simulink model "test_L_detector"  (Simulink 7.6)
settings: Solver=FixedStepDiscrete  StartTime=0.0  StopTime=0  RelTol=1e-3
values from neighbouring files (symbols this model uses):
  Forward_Camera_Dimensions = [640 480]    [VisionConstants.m]
  Iter_Segment_Thresh = 60    [VisionConstants.m]
  Scale_Forward_B = 1    [VisionConstants.m]
  Scale_Forward_G = 1    [VisionConstants.m]
  Scale_Forward_H = .8    (= 0.8)    [VisionConstants.m]
  Scale_Forward_R = 1    [VisionConstants.m]
  Scale_Forward_S = 1    [VisionConstants.m]
  Scale_Forward_V = 2    [VisionConstants.m]
undefined symbols (not defined in the file or in its folder): black_al, black_au, black_bl, black_bu, blue_al, blue_au, blue_bl, blue_bu, Forward_Fov, gray, green_al, green_au, green_bl, green_bu, orange_al, orange_au, orange_bl, orange_bu, Rec, red_al, red_au, red_bl, red_bu, SDTV, white_al, white_au, white_bl, white_bu, yellow_al, yellow_au, yellow_bl, yellow_bu
libraries: vipconversions x4, vipgeotforms x3, viptextngfix x2, vipsnks x2, viptransforms x2, vipanalysis x1, vipsrcs x1
(part 1 of 2)
settings Model: Creator=Thing 1  LastModifiedBy=auvt
settings RTWCC: TargetLang=C++

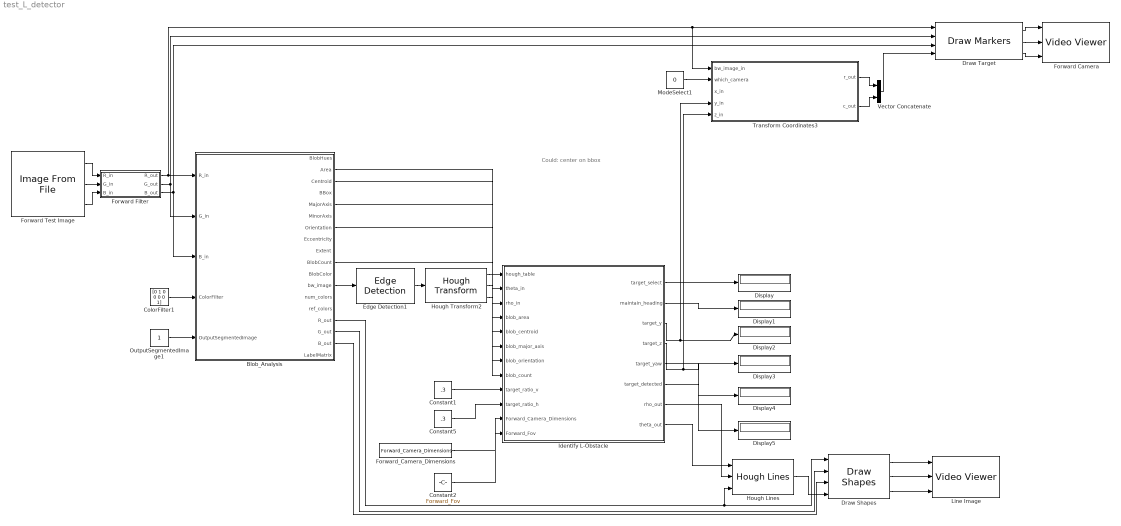
== system test_L_detector ==
  note: Could: center on bbox
  Blob_Analysis : Subsystem
  ColorFilter1 : Constant  Value=[0 1 0 0 0 0 1]  SampleTime=-1
  Constant1 : Constant  Value=.3  SampleTime=-1
  Constant2 : Constant  Value=Forward_Fov  SampleTime=-1
  Constant5 : Constant  Value=.3  SampleTime=-1
  Display{,1..5} (6 alike) : Display
  Draw Shapes : viptextngfix/Draw Shapes  DialogController=vipDDGCreate  DialogControllerArgs=DataTag3  shape=Lines  fill=off  fillClrSource=Specify via dialog  display=Black  intensity=200  color=[200 255 100]  opacity=0.6  viewport=Entire image  antialiasing=off  inType=Obsolete  imagePorts=Separate color signals  prodOutputMode=Binary point scaling  prodOutputWordLength=32  prodOutputFracLength=14  memoryMode=Specify word length  memoryWordLength=16  memoryFracLength=15  roundingMode=Floor  overflowMode=off
  Draw Target : viptextngfix/Draw Markers  DialogController=vipDDGCreate  DialogControllerArgs=DataTag4  shape=X-mark  size=7  fill=off  fillClrSource=Specify via dialog  display=User-specified value  intensity=200  color=[1 0 0]  opacity=0.6  viewport=Entire image  antialiasing=off  inType=Obsolete  imagePorts=Separate color signals  prodOutputMode=Binary point scaling  prodOutputWordLength=32  prodOutputFracLength=14  memoryMode=Specify word length  memoryWordLength=16  memoryFracLength=15  roundingMode=Floor  overflowMode=off
  Edge Detection1 : vipanalysis/Edge Detection  DialogController=vipDDGCreate  DialogControllerArgs=DataTag5  method=Sobel  outputType=Binary image  userDefinedThreshold=off  thresholdSource=Specify via dialog  threshold=20  thresholdTuning=3  edgeThinning=on  threshold_canny=[0.25 0.60]  autoPercent=70  sigma=1  roundingMode=Floor  overflowMode=off
  Forward Camera : vipsnks/Video Viewer  DialogControllerArgs=DataTag7  inputType=Obsolete7b  imagePorts=Separate color signals  useColorMap=off  colormapValue=gray(256)  specRange=off  minInputVal=0  maxInputVal=255  FigPos=[1161 458 276 283]  AxisZoom=on  trueSizedOnce=off  OpenAtMdlStart=on
  Forward Filter : Subsystem
  Forward Test Image : vipsrcs/Image From File  Tag=vipblks_nd  DialogController=vipDDGCreate  DialogControllerArgs=DataTag8  SystemSampleTime=-1  FileName=/home/auvt/auvc/src/vision/Test_Images/L1.PNG  imagePorts=Separate color signals  Ts=-1  ImageDataType=double  Signed=on  WordLength=16  sdImageDataType=uint(8)  FractionLengthMode=User-defined  FractionLength=15  OutPortLabels=R|G|B
  Forward_Camera_Dimensions : Constant  Value=Forward_Camera_Dimensions  SampleTime=-1
  Hough Lines : viptransforms/Hough Lines  DialogController=vipDDGCreate  DialogControllerArgs=DataTag9  sineCompMethod=Trigonometric function  thetaRes=pi/180  firstCoeffMode=Specify word length  firstCoeffWordLength=16  firstCoeffFracLength=15  prodOutputMode=Binary point scaling  prodOutputWordLength=32  prodOutputFracLength=16  roundingMode=Nearest  overflowMode=on
  Hough Transform2 : viptransforms/Hough Transform  DialogController=vipDDGCreate  DialogControllerArgs=DataTag10  theta_res=pi/180  rho_res=1  out_theta_rho=on  outdtmode=double  firstCoeffMode=Binary point scaling  firstCoeffWordLength=16  firstCoeffFracLength=14  secondCoeffMode=Binary point scaling  secondCoeffWordLength=32  secondCoeffFracLength=16  outputMode=Binary point scaling  outputWordLength=16  outputFracLength=0  accumMode=Binary point scaling  accumWordLength=32  accumFracLength=20  prodOutputMode=Binary point scaling  prodOutputWordLength=32  prodOutputFracLength=20  memoryMode=Binary point scaling  memoryWordLength=32  memoryFracLength=16  roundingMode=Nearest  overflowMode=on
  Identify L-Obstacle : Stateflow chart  TreatAsAtomicUnit=on  SystemSampleTime=[1/30 0]
  Line Image : vipsnks/Video Viewer  DialogControllerArgs=DataTag12  inputType=Obsolete7b  imagePorts=Separate color signals  useColorMap=off  colormapValue=gray(256)  specRange=off  minInputVal=0  maxInputVal=255  FigPos=[1163 861 274 294]  AxisZoom=on  trueSizedOnce=off  OpenAtMdlStart=on
  ModeSelect1 : Constant  Value=0  SampleTime=-1
  OutputSegmentedImage1 : Constant  SampleTime=-1
  Transform Coordinates3 : Stateflow chart  TreatAsAtomicUnit=on  SystemSampleTime=[1/30 0]
  Vector Concatenate : Concatenate  Mode=Multidimensional array
  wires:
  Forward Test Image/1 -> Forward Filter/1(R_in)
  Forward Test Image/3 -> Forward Filter/3(B_in)
  Vector Concatenate/1 -> Draw Target/4
  Draw Target/2 -> Forward Camera/2
  Draw Target/1 -> Forward Camera/1
  Draw Target/3 -> Forward Camera/3
  Forward Filter/1(R_out) -> Draw Target/1, Transform Coordinates3/1(bw_image_in), Blob_Analysis/1(R_in)
  Forward Filter/2(G_out) -> Draw Target/2, Blob_Analysis/2(G_in)
  Forward Filter/3(B_out) -> Draw Target/3, Blob_Analysis/3(B_in)
  Forward Test Image/2 -> Forward Filter/2(G_in)
  ModeSelect1/1 -> Transform Coordinates3/2(which_camera)
  Transform Coordinates3/1(r_out) -> Vector Concatenate/1
  Transform Coordinates3/2(c_out) -> Vector Concatenate/2
  OutputSegmentedImage1/1 -> Blob_Analysis/5(OutputSegmentedImage)
  ColorFilter1/1 -> Blob_Analysis/4(ColorFilter)
  Edge Detection1/1 -> Hough Transform2/1
  Blob_Analysis/12(bw_image) -> Edge Detection1/1
  Hough Transform2/1 -> Identify L-Obstacle/1(hough_table)
  Hough Transform2/2 -> Identify L-Obstacle/2(theta_in)
  Hough Transform2/3 -> Identify L-Obstacle/3(rho_in)
  Blob_Analysis/2(Area) -> Identify L-Obstacle/4(blob_area)
  Blob_Analysis/3(Centroid) -> Identify L-Obstacle/5(blob_centroid)
  Blob_Analysis/5(MajorAxis) -> Identify L-Obstacle/6(blob_major_axis)
  Blob_Analysis/7(Orientation) -> Identify L-Obstacle/7(blob_orientation)
  Blob_Analysis/10(BlobCount) -> Identify L-Obstacle/8(blob_count)
  Constant1/1 -> Identify L-Obstacle/9(target_ratio_v)
  Constant5/1 -> Identify L-Obstacle/10(target_ratio_h)
  Forward_Camera_Dimensions/1 -> Identify L-Obstacle/11(Forward_Camera_Dimensions)
  Constant2/1 -> Identify L-Obstacle/12(Forward_Fov)
  Identify L-Obstacle/3(target_y) -> Display2/1, Transform Coordinates3/4(y_in)
  Identify L-Obstacle/1(target_select) -> Display/1
  Identify L-Obstacle/2(maintain_heading) -> Display1/1
  Identify L-Obstacle/4(target_z) -> Display3/1, Transform Coordinates3/5(z_in)
  Identify L-Obstacle/5(target_yaw) -> Display4/1
  Identify L-Obstacle/6(target_detected) -> Display5/1
  Draw Shapes/1 -> Line Image/1
  Draw Shapes/2 -> Line Image/2
  Draw Shapes/3 -> Line Image/3
  Hough Lines/1 -> Draw Shapes/4
  Blob_Analysis/15(R_out) -> Draw Shapes/1, Hough Lines/3
  Blob_Analysis/16(G_out) -> Draw Shapes/2
  Blob_Analysis/17(B_out) -> Draw Shapes/3
  Identify L-Obstacle/8(theta_out) -> Hough Lines/1
  Identify L-Obstacle/7(rho_out) -> Hough Lines/2

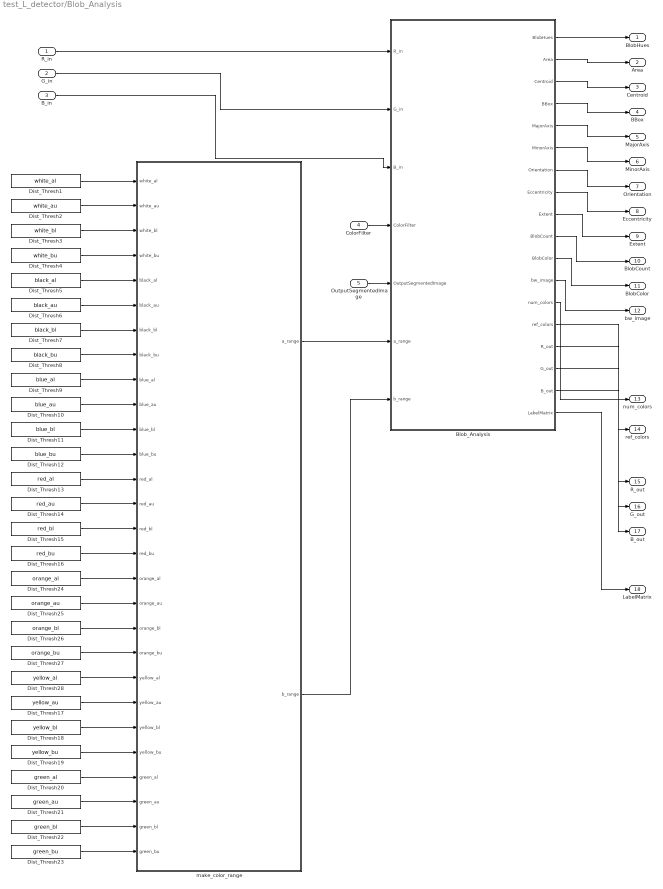
== system test_L_detector/Blob_Analysis ==
  R_in : Inport
  G_in : Inport  Port=2
  B_in : Inport  Port=3
  ColorFilter : Inport  Port=4
  OutputSegmentedImage : Inport  Port=5
  Blob_Analysis : Subsystem  TreatAsAtomicUnit=on
  Dist_Thresh1 : Constant  Value=white_al  SampleTime=-1
  Dist_Thresh10 : Constant  Value=blue_au  SampleTime=-1
  Dist_Thresh11 : Constant  Value=blue_bl  SampleTime=-1
  Dist_Thresh12 : Constant  Value=blue_bu  SampleTime=-1
  Dist_Thresh13 : Constant  Value=red_al  SampleTime=-1
  Dist_Thresh14 : Constant  Value=red_au  SampleTime=-1
  Dist_Thresh15 : Constant  Value=red_bl  SampleTime=-1
  Dist_Thresh16 : Constant  Value=red_bu  SampleTime=-1
  Dist_Thresh17 : Constant  Value=yellow_au  SampleTime=-1
  Dist_Thresh18 : Constant  Value=yellow_bl  SampleTime=-1
  Dist_Thresh19 : Constant  Value=yellow_bu  SampleTime=-1
  Dist_Thresh2 : Constant  Value=white_au  SampleTime=-1
  Dist_Thresh20 : Constant  Value=green_al  SampleTime=-1
  Dist_Thresh21 : Constant  Value=green_au  SampleTime=-1
  Dist_Thresh22 : Constant  Value=green_bl  SampleTime=-1
  Dist_Thresh23 : Constant  Value=green_bu  SampleTime=-1
  Dist_Thresh24 : Constant  Value=orange_al  SampleTime=-1
  Dist_Thresh25 : Constant  Value=orange_au  SampleTime=-1
  Dist_Thresh26 : Constant  Value=orange_bl  SampleTime=-1
  Dist_Thresh27 : Constant  Value=orange_bu  SampleTime=-1
  Dist_Thresh28 : Constant  Value=yellow_al  SampleTime=-1
  Dist_Thresh3 : Constant  Value=white_bl  SampleTime=-1
  Dist_Thresh4 : Constant  Value=white_bu  SampleTime=-1
  Dist_Thresh5 : Constant  Value=black_al  SampleTime=-1
  Dist_Thresh6 : Constant  Value=black_au  SampleTime=-1
  Dist_Thresh7 : Constant  Value=black_bl  SampleTime=-1
  Dist_Thresh8 : Constant  Value=black_bu  SampleTime=-1
  Dist_Thresh9 : Constant  Value=blue_al  SampleTime=-1
  make_color_range : Stateflow chart  TreatAsAtomicUnit=on
  BlobHues : Outport
  Area : Outport  Port=2
  Centroid : Outport  Port=3
  BBox : Outport  Port=4
  MajorAxis : Outport  Port=5
  MinorAxis : Outport  Port=6
  Orientation : Outport  Port=7
  Eccentricity : Outport  Port=8
  Extent : Outport  Port=9
  BlobCount : Outport  Port=10
  BlobColor : Outport  Port=11
  bw_image : Outport  Port=12
  num_colors : Outport  Port=13
  ref_colors : Outport  Port=14
  R_out : Outport  Port=15
  G_out : Outport  Port=16
  B_out : Outport  Port=17
  LabelMatrix : Outport  Port=18
  wires:
  Dist_Thresh23/1 -> make_color_range/28(green_bu)
  Dist_Thresh22/1 -> make_color_range/27(green_bl)
  Dist_Thresh1/1 -> make_color_range/1(white_al)
  Dist_Thresh18/1 -> make_color_range/23(yellow_bl)
  Dist_Thresh19/1 -> make_color_range/24(yellow_bu)
  Dist_Thresh20/1 -> make_color_range/25(green_al)
  Dist_Thresh17/1 -> make_color_range/22(yellow_au)
  Dist_Thresh28/1 -> make_color_range/21(yellow_al)
  Dist_Thresh21/1 -> make_color_range/26(green_au)
  Dist_Thresh27/1 -> make_color_range/20(orange_bu)
  Dist_Thresh26/1 -> make_color_range/19(orange_bl)
  Dist_Thresh25/1 -> make_color_range/18(orange_au)
  Dist_Thresh24/1 -> make_color_range/17(orange_al)
  Dist_Thresh16/1 -> make_color_range/16(red_bu)
  Dist_Thresh15/1 -> make_color_range/15(red_bl)
  Dist_Thresh14/1 -> make_color_range/14(red_au)
  Dist_Thresh13/1 -> make_color_range/13(red_al)
  Dist_Thresh12/1 -> make_color_range/12(blue_bu)
  Dist_Thresh11/1 -> make_color_range/11(blue_bl)
  Dist_Thresh10/1 -> make_color_range/10(blue_au)
  Dist_Thresh9/1 -> make_color_range/9(blue_al)
  Dist_Thresh8/1 -> make_color_range/8(black_bu)
  Dist_Thresh2/1 -> make_color_range/2(white_au)
  Dist_Thresh3/1 -> make_color_range/3(white_bl)
  Dist_Thresh4/1 -> make_color_range/4(white_bu)
  Dist_Thresh5/1 -> make_color_range/5(black_al)
  Dist_Thresh6/1 -> make_color_range/6(black_au)
  Dist_Thresh7/1 -> make_color_range/7(black_bl)
  R_in/1 -> Blob_Analysis/1(R_in)
  G_in/1 -> Blob_Analysis/2(G_in)
  B_in/1 -> Blob_Analysis/3(B_in)
  make_color_range/1(a_range) -> Blob_Analysis/6(a_range)
  make_color_range/2(b_range) -> Blob_Analysis/7(b_range)
  OutputSegmentedImage/1 -> Blob_Analysis/5(OutputSegmentedImage)
  ColorFilter/1 -> Blob_Analysis/4(ColorFilter)
  Blob_Analysis/1(BlobHues) -> BlobHues/1
  Blob_Analysis/2(Area) -> Area/1
  Blob_Analysis/3(Centroid) -> Centroid/1
  Blob_Analysis/4(BBox) -> BBox/1
  Blob_Analysis/5(MajorAxis) -> MajorAxis/1
  Blob_Analysis/6(MinorAxis) -> MinorAxis/1
  Blob_Analysis/7(Orientation) -> Orientation/1
  Blob_Analysis/8(Eccentricity) -> Eccentricity/1
  Blob_Analysis/9(Extent) -> Extent/1
  Blob_Analysis/10(BlobCount) -> BlobCount/1
  Blob_Analysis/11(BlobColor) -> BlobColor/1
  Blob_Analysis/12(bw_image) -> bw_image/1
  Blob_Analysis/13(num_colors) -> num_colors/1
  Blob_Analysis/14(ref_colors) -> ref_colors/1
  Blob_Analysis/15(R_out) -> R_out/1
  Blob_Analysis/16(G_out) -> G_out/1
  Blob_Analysis/17(B_out) -> B_out/1
  Blob_Analysis/18(LabelMatrix) -> LabelMatrix/1

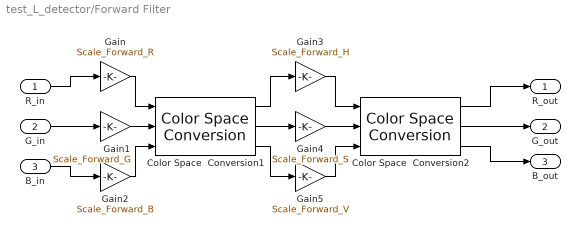
== system test_L_detector/Forward Filter ==
  R_in : Inport  PortDimensions=Forward_Camera_Dimensions
  G_in : Inport  Port=2  PortDimensions=Forward_Camera_Dimensions
  B_in : Inport  Port=3  PortDimensions=Forward_Camera_Dimensions
  Color Space  Conversion1 : vipconversions/Color Space  Conversion  conversion=Obsolete  conversionActive=R'G'B' to HSV  wp_str=D50  rec=Rec. 601 (SDTV)  sys=1125/60/2:1  imagePorts=Separate color signals
  Color Space  Conversion2 : vipconversions/Color Space  Conversion  conversion=Obsolete  conversionActive=HSV to R'G'B'  wp_str=D50  rec=Rec. 601 (SDTV)  sys=1125/60/2:1  imagePorts=Separate color signals
  Gain : Gain  Gain=Scale_Forward_R
  Gain1 : Gain  Gain=Scale_Forward_G
  Gain2 : Gain  Gain=Scale_Forward_B
  Gain3 : Gain  Gain=Scale_Forward_H
  Gain4 : Gain  Gain=Scale_Forward_S
  Gain5 : Gain  Gain=Scale_Forward_V
  R_out : Outport  OutDataTypeStr=double
  G_out : Outport  Port=2  OutDataTypeStr=double
  B_out : Outport  Port=3  OutDataTypeStr=double
  wires:
  R_in/1 -> Gain/1
  G_in/1 -> Gain1/1
  B_in/1 -> Gain2/1
  Gain/1 -> Color Space  Conversion1/1
  Gain1/1 -> Color Space  Conversion1/2
  Gain2/1 -> Color Space  Conversion1/3
  Color Space  Conversion1/1 -> Gain3/1
  Color Space  Conversion1/2 -> Gain4/1
  Color Space  Conversion1/3 -> Gain5/1
  Gain3/1 -> Color Space  Conversion2/1
  Gain4/1 -> Color Space  Conversion2/2
  Gain5/1 -> Color Space  Conversion2/3
  Color Space  Conversion2/1 -> R_out/1
  Color Space  Conversion2/2 -> G_out/1
  Color Space  Conversion2/3 -> B_out/1

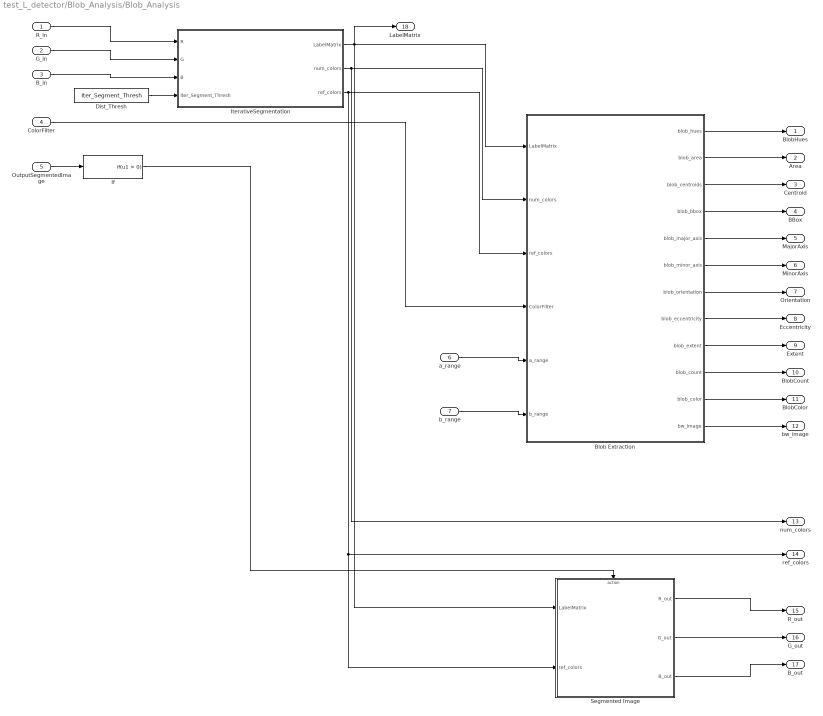
== system test_L_detector/Blob_Analysis/Blob_Analysis ==
  R_in : Inport
  G_in : Inport  Port=2
  B_in : Inport  Port=3
  ColorFilter : Inport  Port=4
  OutputSegmentedImage : Inport  Port=5
  a_range : Inport  Port=6
  b_range : Inport  Port=7
  Blob Extraction : Stateflow chart  TreatAsAtomicUnit=on
  Dist_Thresh : Constant  Value=Iter_Segment_Thresh  SampleTime=-1
  If : If  ShowElse=off
  IterativeSegmentation : Subsystem
      settings: UndoDeleteFcn=Stateflow.SLINSF.SimulinkMan.restorePreDeleteFcn  PreDeleteFcn=Stateflow.SLINSF.SimulinkMan.removePreDeleteFcn
  Segmented Image : Subsystem  TreatAsAtomicUnit=on
  BlobHues : Outport
  Area : Outport  Port=2
  Centroid : Outport  Port=3
  BBox : Outport  Port=4
  MajorAxis : Outport  Port=5
  MinorAxis : Outport  Port=6
  Orientation : Outport  Port=7
  Eccentricity : Outport  Port=8
  Extent : Outport  Port=9
  BlobCount : Outport  Port=10
  BlobColor : Outport  Port=11
  bw_image : Outport  Port=12
  num_colors : Outport  Port=13
  ref_colors : Outport  Port=14
  R_out : Outport  Port=15
  G_out : Outport  Port=16
  B_out : Outport  Port=17
  LabelMatrix : Outport  Port=18
  wires:
  Blob Extraction/12(bw_image) -> bw_image/1
  Blob Extraction/10(blob_count) -> BlobCount/1
  Blob Extraction/9(blob_extent) -> Extent/1
  Blob Extraction/8(blob_eccentricity) -> Eccentricity/1
  Blob Extraction/7(blob_orientation) -> Orientation/1
  Blob Extraction/6(blob_minor_axis) -> MinorAxis/1
  Blob Extraction/5(blob_major_axis) -> MajorAxis/1
  Blob Extraction/4(blob_bbox) -> BBox/1
  Blob Extraction/3(blob_centroids) -> Centroid/1
  Blob Extraction/2(blob_area) -> Area/1
  Blob Extraction/1(blob_hues) -> BlobHues/1
  ColorFilter/1 -> Blob Extraction/4(ColorFilter)
  a_range/1 -> Blob Extraction/5(a_range)
  b_range/1 -> Blob Extraction/6(b_range)
  IterativeSegmentation/1(LabelMatrix) -> Blob Extraction/1(LabelMatrix), Segmented Image/1(LabelMatrix), LabelMatrix/1
  IterativeSegmentation/2(num_colors) -> Blob Extraction/2(num_colors), num_colors/1
  IterativeSegmentation/3(ref_colors) -> Blob Extraction/3(ref_colors), Segmented Image/2(ref_colors), ref_colors/1
  Dist_Thresh/1 -> IterativeSegmentation/4(Iter_Segment_Thresh)
  R_in/1 -> IterativeSegmentation/1(R)
  G_in/1 -> IterativeSegmentation/2(G)
  B_in/1 -> IterativeSegmentation/3(B)
  If/1 -> Segmented Image/Action
  OutputSegmentedImage/1 -> If/1
  Segmented Image/1(R_out) -> R_out/1
  Segmented Image/2(G_out) -> G_out/1
  Segmented Image/3(B_out) -> B_out/1
  Blob Extraction/11(blob_color) -> BlobColor/1

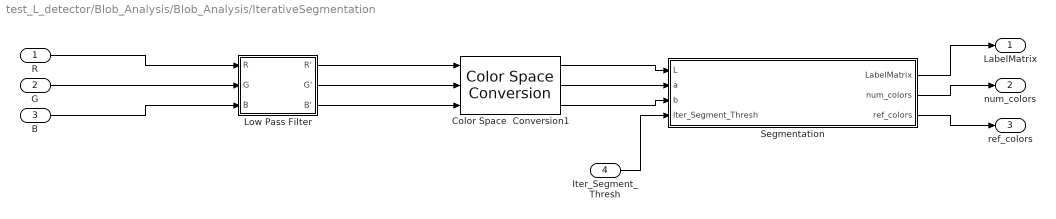
== system test_L_detector/Blob_Analysis/Blob_Analysis/IterativeSegmentation ==
  R : Inport
  G : Inport  Port=2
  B : Inport  Port=3
  Iter_Segment_Thresh : Inport  Port=4
  Color Space  Conversion1 : vipconversions/Color Space  Conversion  conversion=Obsolete  conversionActive=sR'G'B' to L*a*b*  wp_str=D50  rec=Rec. 601 (SDTV)  sys=1125/60/2:1  imagePorts=Separate color signals
  Low Pass Filter : Subsystem
  Segmentation : Subsystem
  LabelMatrix : Outport
  num_colors : Outport  Port=2
  ref_colors : Outport  Port=3
  wires:
  Low Pass Filter/3(B') -> Color Space  Conversion1/3
  Low Pass Filter/2(G') -> Color Space  Conversion1/2
  Low Pass Filter/1(R') -> Color Space  Conversion1/1
  Color Space  Conversion1/3 -> Segmentation/3(b)
  Color Space  Conversion1/2 -> Segmentation/2(a)
  Color Space  Conversion1/1 -> Segmentation/1(L)
  R/1 -> Low Pass Filter/1(R)
  G/1 -> Low Pass Filter/2(G)
  B/1 -> Low Pass Filter/3(B)
  Segmentation/1(LabelMatrix) -> LabelMatrix/1
  Segmentation/2(num_colors) -> num_colors/1
  Segmentation/3(ref_colors) -> ref_colors/1
  Iter_Segment_Thresh/1 -> Segmentation/4(Iter_Segment_Thresh)

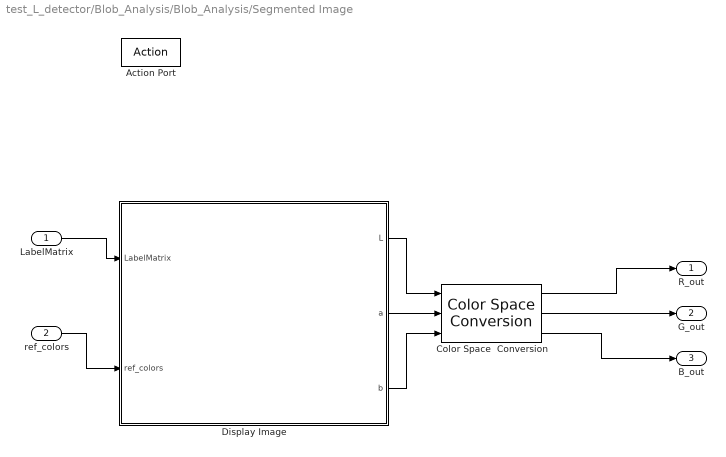
== system test_L_detector/Blob_Analysis/Blob_Analysis/Segmented Image ==
  LabelMatrix : Inport
  ref_colors : Inport  Port=2
  Action Port : ActionPort  ActionType=then
  Color Space  Conversion : vipconversions/Color Space  Conversion  conversion=Obsolete  conversionActive=L*a*b* to sR'G'B'  wp_str=D65  rec=Rec. 601 (SDTV)  sys=1125/60/2:1  imagePorts=Separate color signals
  Display Image : Stateflow chart  TreatAsAtomicUnit=on
  R_out : Outport
  G_out : Outport  Port=2
  B_out : Outport  Port=3
  wires:
  LabelMatrix/1 -> Display Image/1(LabelMatrix)
  ref_colors/1 -> Display Image/2(ref_colors)
  Display Image/1(L) -> Color Space  Conversion/1
  Display Image/2(a) -> Color Space  Conversion/2
  Display Image/3(b) -> Color Space  Conversion/3
  Color Space  Conversion/1 -> R_out/1
  Color Space  Conversion/2 -> G_out/1
  Color Space  Conversion/3 -> B_out/1

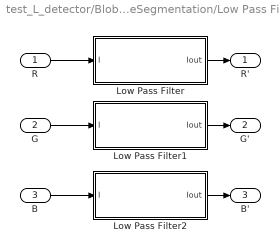
== system test_L_detector/Blob_Analysis/Blob_Analysis/IterativeSegmentation/Low Pass Filter ==
  R : Inport
  G : Inport  Port=2
  B : Inport  Port=3
  Low Pass Filter : Stateflow chart  TreatAsAtomicUnit=on
  Low Pass Filter1 : Stateflow chart  TreatAsAtomicUnit=on
  Low Pass Filter2 : Stateflow chart  TreatAsAtomicUnit=on
  R' : Outport
  G' : Outport  Port=2
  B' : Outport  Port=3
  wires:
  Low Pass Filter/1(Iout) -> R'/1
  Low Pass Filter2/1(Iout) -> B'/1
  Low Pass Filter1/1(Iout) -> G'/1
  B/1 -> Low Pass Filter2/1(I)
  G/1 -> Low Pass Filter1/1(I)
  R/1 -> Low Pass Filter/1(I)

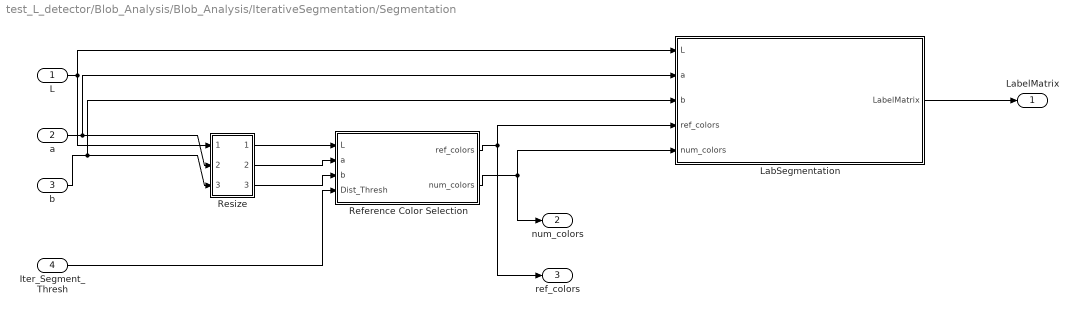
== system test_L_detector/Blob_Analysis/Blob_Analysis/IterativeSegmentation/Segmentation ==
  L : Inport
  a : Inport  Port=2
  b : Inport  Port=3
  Iter_Segment_Thresh : Inport  Port=4
  LabSegmentation : Stateflow chart  TreatAsAtomicUnit=on
  Reference Color Selection : Stateflow chart  TreatAsAtomicUnit=on
  Resize : Subsystem
  LabelMatrix : Outport
  num_colors : Outport  Port=2
  ref_colors : Outport  Port=3
  wires:
  Iter_Segment_Thresh/1 -> Reference Color Selection/4(Dist_Thresh)
  LabSegmentation/1(LabelMatrix) -> LabelMatrix/1
  Reference Color Selection/2(num_colors) -> LabSegmentation/5(num_colors), num_colors/1
  Reference Color Selection/1(ref_colors) -> ref_colors/1, LabSegmentation/4(ref_colors)
  Resize/3(Out3) -> Reference Color Selection/3(b)
  Resize/2(Out2) -> Reference Color Selection/2(a)
  Resize/1(Out1) -> Reference Color Selection/1(L)
  b/1 -> LabSegmentation/3(b), Resize/3(In3)
  a/1 -> LabSegmentation/2(a), Resize/2(In2)
  L/1 -> LabSegmentation/1(L), Resize/1(In1)

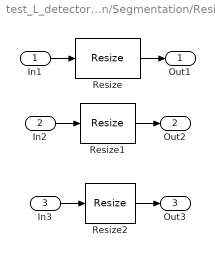
== system test_L_detector/Blob_Analysis/Blob_Analysis/IterativeSegmentation/Segmentation/Resize ==
  In1 : Inport
  In2 : Inport  Port=2
  In3 : Inport  Port=3
  Resize : vipgeotforms/Resize  DialogController=vipDDGCreate  DialogControllerArgs=DataTag0  specify=Number of output rows and columns  rfactor=[]  outCols=25  outRows=25  outRowsCols=[60 80]  interp_method=Bilinear  antialias=on  useROI=off  roiFlag=off  prodOutputMode=Binary point scaling  prodOutputWordLength=32  prodOutputFracLength=10  roundingMode=Nearest  overflowMode=on
  Resize1 : vipgeotforms/Resize  DialogController=vipDDGCreate  DialogControllerArgs=DataTag1  specify=Number of output rows and columns  rfactor=[200 150]  outCols=25  outRows=25  outRowsCols=[60 80]  interp_method=Bilinear  antialias=on  useROI=off  roiFlag=off  prodOutputMode=Binary point scaling  prodOutputWordLength=32  prodOutputFracLength=10  roundingMode=Nearest  overflowMode=on
  Resize2 : vipgeotforms/Resize  DialogController=vipDDGCreate  DialogControllerArgs=DataTag2  specify=Number of output rows and columns  rfactor=[200 150]  outCols=25  outRows=25  outRowsCols=[60 80]  interp_method=Bilinear  antialias=on  useROI=off  roiFlag=off  prodOutputMode=Binary point scaling  prodOutputWordLength=32  prodOutputFracLength=10  roundingMode=Nearest  overflowMode=on
  Out1 : Outport
  Out2 : Outport  Port=2
  Out3 : Outport  Port=3
  wires:
  Resize2/1 -> Out3/1
  In3/1 -> Resize2/1
  Resize1/1 -> Out2/1
  In2/1 -> Resize1/1
  Resize/1 -> Out1/1
  In1/1 -> Resize/1

== matlab function Transform Coordinates3 ==
  data: bw_image_in input double; which_camera input double; x_in input double; y_in input double; r_out output double; c_out output double; z_in input double
function [r_out, c_out] = transform_G2L(bw_image_in, which_camera, x_in, y_in, z_in)
% This function, "transform Global to Local coordinates," transforms
%   global coordinates that are sent to the controller into local
%   coordinates that can be displayed over images.
%
% 5-29-11
%
% Input
%   x_in, y_in, z_in = vectors of points in global (vehicle-centered)
%     coordinate system
%   bw_image_in = a 2-D array of pixel values (used only to extract image
%     size)
%   which_camera = selects which camera for relative coordinates
%                = 0 -> Forward camera
%                = 1 -> Down camera
%
% Output
%   r_out, c_out = row, column pairs in local coordinate system

[rows, cols] = size(bw_image_in);
if( which_camera == 0 )
    r_out = z_in + floor(rows/2);
    c_out = y_in + floor(cols/2);
else
    r_out = floor(rows/2) - x_in;
    c_out = y_in + floor(cols/2);
end

return

== matlab function Identify L-Obstacle ==
  data: target_select output double; maintain_heading output double; hough_table input double; target_y output double; target_z output double; target_yaw output double; target_detected output double; theta_in input double; rho_in input double; blob_area input double; blob_centroid input double; blob_major_axis input double; blob_orientation input double; blob_count input double; target_ratio_v input double; target_ratio_h input double; Forward_Camera_Dimensions input double; Forward_Fov input double; rho_out output double; theta_out output double
function [target_select, maintain_heading, target_y, target_z, target_yaw, target_detected,  rho_out, theta_out] = validation_gate(hough_table, theta_in, rho_in, blob_area, blob_centroid, blob_major_axis, blob_orientation, blob_count, target_ratio_v, target_ratio_h, Forward_Camera_Dimensions, Forward_Fov)
%#eml
%{

1. Iteratively segment image
2. Obtain information about all blobs in image
3. Generate a bw image by filtering colors (thresholding)

3.5. Identify one appropriate horizontal and one appropriate vertical blob

4. Perform edge detection then Hough transform to bw image
5. Identify the most popular lines (any orientation) that are:
     a) Nearly colinear with blobs, and
     b) At approximately 90 degrees from each other

6. Target appropriately

%}




% This function attempts to identfiy the L-shaped obstacle, and returns
%   targeting information, and a true/false target_detected parameter.


% Initialize
target_select = 1;
maintain_heading = 0;
target_y = 0;
target_z = 0;
target_yaw = 0;
target_detected = 0;


% Only the (max_num_lines) with the most votes will be considered as
%   candidates for the gate
max_num_lines = 200;
[rho_length, theta_length] = size(hough_table);
rows = Forward_Camera_Dimensions(1);
cols = Forward_Camera_Dimensions(2);

image_area = rows*cols;
area_thresh = 0.8;  % Ratio of blob area to image area considered to imply the blob is actually background noise

% eps_rho must be at least as big as the gate leg diameter (units of
%   pixels)
eps_rho = .1*max(rows,cols);
% eps_theta is used to distinguish lines as "horizontal" or "vertical";
%   units are radians
eps_theta = 10*pi/180;

% These vectors contain the final two lines that compose the L-obstacle
rho_gate = zeros(1,2);
theta_gate = zeros(1,2);

% These vectors contain intermediate line information; as lines are
%   eliminated from these vectors, their values are set to zero
% Note that rho_in and theta_in are referred to by hough_table; they do not
%   constitute (rho,theta) pairs without hough_table. rho and therhota,
%   however, do constitute (rho,theta) pairs.
rho = zeros(1,max_num_lines);
theta = zeros(1,max_num_lines);


% Identify the most popular max_num_lines lines
i_index = ones(1,max_num_lines);
j_index = ones(1,max_num_lines);

for m = 1:max_num_lines
    
    max_votes = 0;
    for i = 1:rho_length
        for j = 1:theta_length
            if( hough_table(i,j) > max_votes )
                i_index(m) = i;
                j_index(m) = j;
                max_votes = hough_table(i,j);
            end
        end
    end
    
    rho(m) = rho_in(i_index(m));
    theta(m) = theta_in(j_index(m));
    hough_table(i_index(m),j_index(m)) = 0;
    
end


% Correct orientations to vehicle coordinates
for j = 1:blob_count
    % theta_hold:
    %   -is between [-pi/2, +pi/2]
    % blob_orientation:
    %   -is potentially outside this range
    %   -needs to be corrected by pi/2 to get relative heading
    blob_orientation(j) = mod(pi - blob_orientation(j), pi) - pi/2;
end


% Determine the most popular lines which are nearly colinear to blobs
theta_hold = theta;
i_gate = zeros(2,2);  % Indices for line and blob, respectively
for g = 1:2
    
    found = 0;
    for i = 1:max_num_lines
        for j = 1:blob_count
            
            % Search for a match between one blob and one line
            condition1 = abs(theta_hold(i) - blob_orientation(j)) <= eps_theta;
            condition2 = blob_area(j)/image_area <= area_thresh;
            condition3 = theta_hold(i) ~= 1000 && blob_orientation(j) ~= 1000;
            c1 = blob_centroid(2,j);
            r1 = blob_centroid(1,j);
            c2 = rho(i)*cos(theta_hold(i)) - r1 + c1*sin(theta_hold(i));
            r2 = -cot(theta_hold(i))*c2 + rho(i)/sin(theta_hold(i));
%            c2 = rho(i)*cos(theta(i)) - r1 + c1*sin(theta(i));
%            r2 = -cot(theta(i))*c2 + rho(i)/sin(theta(i));
            d = sqrt( (c2 - c1)^2 + (r2 - r1)^2 );
            condition4 = d <= eps_rho;
            if(condition1 && condition2 && condition3 && condition4)
                
                if(g == 1)
                    
                    % Determine the first gate element
                    i_gate(1,g) = i;
                    i_gate(2,g) = j;
                    
                else
                    
                    % Assume the first gate element was found correctly;
                    %   check that all other gate elements are at right
                    %   angles to the first
                    if( abs((pi/2) - abs(theta_hold(i) - theta_hold( i_gate(1,1) ))) <= eps_theta)
                        i_gate(1,g) = i;
                        i_gate(2,g) = j;
                    end
                    
                end
                
                theta_hold(i) = 1000;  % Invalid angle; do not want this line to be selected again
                blob_orientation(j) = 1000;
                found = 1;
                break;
            end
            
        end
        
        if(found == 1)
            break;
        end
    end
    
end





rho_out = zeros(1,max_num_lines);
theta_out = zeros(1,max_num_lines);

%rho_out( i_gate(1,1) ) = rho( i_gate(1,1) );
%theta_out( i_gate(1,1) ) = theta_out( i_gate(1,1) );
%rho_out( i_gate(1,2) ) = rho( i_gate(1,2) );
%theta_out( i_gate(1,2) ) = theta_out( i_gate(1,2) );




if( ~(i_gate(1) == 0 && i_gate(2) == 0) )
    
    % Sort elements of i_gate to place the vertical element in the first
    %   position, horizontal element in second position
    ihold = i_gate(1,1);
    jhold = i_gate(2,1);
    if( abs(theta( i_gate(1,1) )) > abs(theta( i_gate(1,2) )) )
        i_gate(1,1) = i_gate(1,2);
        i_gate(2,1) = i_gate(2,2);

        i_gate(1,2) = ihold;
        i_gate(2,2) = jhold;
    end


    % Assign appropriate gate information
    for g = 1:2
        rho_gate(g) = rho( i_gate(1,g) );
        theta_gate(g) = theta( i_gate(1,g) );
    end


    % Compute targeting information
    % Determine side lengths and distances for target
    length1 = blob_major_axis(i_gate(2,1));
    length2 = blob_major_axis(i_gate(2,2));
    d1 = target_ratio_v*length1;
    d2 = target_ratio_h*length2;

    phi1 = blob_orientation(i_gate(2,1));
    phi2 = blob_orientation(i_gate(2,2));
    theta1 = (pi/2) - phi1;
    theta2 = (pi/2) - phi2;

    r1 = blob_centroid(1,i_gate(2,1));
    c1 = blob_centroid(2,i_gate(2,1));
    r2 = blob_centroid(1,i_gate(2,2));
    c2 = blob_centroid(2,i_gate(2,2));

    rho1 = c1*sin(theta1) + r1*cos(theta1);
    rho2 = c2*sin(theta2) + r2*cos(theta2);

    r3 = (1/( cos(theta1)*sin(theta2) - cos(theta2)*sin(theta1) ))*( rho1*sin(theta2) - rho2*sin(theta1) );
    c3 = -cot(theta1)*r3 + rho1/sin(theta1);
    %r3 = (1/( sin(phi1)*cos(phi2) - sin(phi2)*cos(phi1) ))*( c2 - c1 + sin(pih1)*cos(phi2)*r1 - sin(phi2)*cos(phi1)*r2 );
    %c3 = r3*tan(phi1) + c1 - r1*tan(phi1);

    r4 = r3 - d1*cos(phi1);
    c4 = c3 + d1*sin(phi1);

    r5 = r3 + d2*sin(phi2);
    c5 = c3 + d2*cos(phi2);

    theta4 = theta1;
    theta5 = theta2;

    rho4 = c4*sin(theta4) + r4*cos(theta4);
    rho5 = c5*sin(theta5) + r5*cos(theta5);

    r6 = (1/( cos(theta4)*sin(theta5) - cos(theta5)*sin(theta4) ))*( rho4*sin(theta5) - rho5*sin(theta4) );
    c6 = -cot(theta4)*r6 + rho4/sin(theta4);
    
    target_detected = 1;
    
    % Transform target r, c to global coordinate system
    target_z = r6 - floor(rows/2);
    target_y = c6 - floor(cols/2);
    
    target_yaw = Forward_Fov*( target_y/cols );
    target_detected = 0;
    
else
    
    target_y = 0;
    target_z = 0;
    target_yaw = 0;
    target_detected = 0;
    
end


return

== matlab function Blob_Analysis/Blob_Analysis/Blob Extraction ==
  data: LabelMatrix input double; num_colors input double; ref_colors input double; ColorFilter input double; a_range input double; b_range input double; blob_hues output double; blob_area output double; blob_centroids output double; blob_bbox output double; blob_major_axis output double; blob_minor_axis output double; blob_orientation output double; blob_eccentricity output double; blob_extent output double; blob_count output double; blob_color output double; bw_image output double
function [blob_hues, blob_area, blob_centroids, blob_bbox, blob_major_axis, blob_minor_axis, blob_orientation, blob_eccentricity, blob_extent, blob_count, blob_color, bw_image] = GetBlobInfo(LabelMatrix, num_colors, ref_colors, ColorFilter, a_range, b_range)
% This function calculates blob information for each color component after
%   iterative segmentation


% Output
%   blob_color = 1xN vector of color indices (global color scheme)


% Initialize
max_num_blobs = 50;
min_blob_area = 5;

[rows, cols] = size(LabelMatrix);
image_area = rows*cols;
LogicMatrix = false(rows,cols);
bw_image = zeros(rows,cols);

blob_hues = zeros(3,max_num_blobs);
blob_area = -1.*ones(1,max_num_blobs);
blob_bbox = zeros(4,max_num_blobs);
blob_major_axis = zeros(1,max_num_blobs);
blob_minor_axis = zeros(1,max_num_blobs);
blob_centroids = zeros(2,max_num_blobs);
blob_eccentricity = zeros(1,max_num_blobs);
blob_extent = zeros(1,max_num_blobs);
blob_orientation = zeros(1,max_num_blobs);
blob_count = 0;

blob_color = zeros(1,max_num_blobs);

max_num_col_filter = length(ColorFilter);
num_col_filter = sum(ColorFilter);

area_thresh = .1;


% Determine L_white and L_black as needed
find_white = 0;
find_black = 0;
L_white = 101;
L_black = -1;
color_areas = zeros(1,size(ref_colors,1));

if(ColorFilter(1) + ColorFilter(2) > 0)
    for row = 1:rows
        for col = 1:cols
            color_areas(LabelMatrix(row,col)) = color_areas(LabelMatrix(row,col)) + 1;
        end
    end
end

if(ColorFilter(1) == 1)
    
    % Determine the brightest colors, but allow a maximum area
    %   ratio of the image to be "white"
    find_white = 1;
    
    positive_area = 0;
    for n = 1:num_colors
        
        maxL = -1;
        k_max = -1;
        for k = 1:num_colors
            L = ref_colors(k,1);
            if(L > maxL && L < L_white)
                maxL = L;
                k_max = k;
            end
        end
        
        positive_area = positive_area + color_areas(k_max);
        if(positive_area/image_area >= area_thresh && n > 1)
            break;
        end
        
        L_white = maxL;
        
    end
end

if(ColorFilter(2) == 1)
    
    % Determine the darkest colors, but allow a maximum area
    %   ratio of the image to be "black"
    find_black = 1;
    
    for row = 1:rows
        for col = 1:cols
            color_areas(LabelMatrix(row,col)) = color_areas(LabelMatrix(row,col)) + 1;
        end
    end
    
    positive_area = 0;
    for n = 1:num_colors
        
        minL = 101;
        k_min = -1;
        for k = 1:num_colors
            L = ref_colors(k,1);
            if(L < minL && L > L_black)
                minL = L;
                k_min = k;
            end
        end
        
        positive_area = positive_area + color_areas(k_min);
        if(positive_area/image_area >= area_thresh && n > 1)
            break;
        end
        
        L_black = minL;
        
    end
end


% Input hblob, a matrix containing [Area, blob_centroids, Eccentricity] for each
% identified blob
persistent hblob
if isempty(hblob)
    hblob = video.BlobAnalysis('AreaOutputPort',true,'CentroidOutputPort',true,...
        'BoundingBoxOutputPort',true,'MajorAxisLengthOutputPort',true,'MinorAxisLengthOutputPort',true,...
        'OrientationOutputPort',true,...
        'EccentricityOutputPort',true,'ExtentOutputPort',true,'NumBlobsOutputPort',true,...
        'MinimumBlobAreaSource','Property','MinimumBlobArea', min_blob_area);
end


% Calculate geometric information about the blobs
%
% LogicMatrix is a binary version of LabelMatrix, with ones at all
%   locations for which color values are k, and zeros everywhere else
%
% Explanation
%   condition1 == 1 causes the k'th color to be analyzed by blob analysis,
%     as well as be included in the black-and-white image
%   condition1 == 0 disallows both of these items and simply ignores color
%     k
%   condition0 == 1 ensures that condition1 is true for all k
%   condition0 == 0 enforces a filter which allows only the colors
%     specified in the ColorFilter vector
condition0 = (num_col_filter == 0);
current_color = 0;
for k = 1:num_colors
    
    % Decide whether or not to perform blob analysis
    condition1 = 0;
    if(condition0)
        condition1 = 1;
    else
        a = ref_colors(k, 2);
        b = ref_colors(k, 3);
        for i = 1:max_num_col_filter
            
            % Skip colors that have not been specified
            if(ColorFilter(i) == 0)
                continue;
            end
            
            if( find_white == 1 && ref_colors(k,1) >= L_white)  % Handle "white" differently than other colors
                condition1 = 1;
                current_color = 1;
                break;
            elseif( find_black == 1 && ref_colors(k,1) <= L_black)  % Handle "black" differently than other colors
                condition1 = 1;
                current_color = 2;
                break;
            elseif( a >= a_range(1,i) && a <= a_range(2,i) && b >= b_range(1,i) && b <= b_range(2,i) )
                condition1 = 1;
                current_color = i;
                break;
            end
            
        end
    end
    
    % Blob analysis
    if( condition1 == 1 )
        
        for i = 1:rows
            for j = 1:cols
                if(LabelMatrix(i,j) ~= k)
                    LogicMatrix(i,j) = false;
                else
                    LogicMatrix(i,j) = true;
                    bw_image(i,j) = 1;
                end
            end
        end

        [TArea,TCentroid,TBBox,TMajorAxis,TMinorAxis,TOrientation,TEccent,TExtent,TNumBlobs] = step(hblob,LogicMatrix);

        for i = 1:TNumBlobs
            if(blob_count + TNumBlobs <= max_num_blobs)

                blob_centroids(1,blob_count+i) = TCentroid(1,i);
                blob_centroids(2,blob_count+i) = TCentroid(2,i);

                ii = round(blob_centroids(1,blob_count+i));
                jj = round(blob_centroids(2,blob_count+i));

                blob_hues(1,blob_count+i) = ref_colors( LabelMatrix(ii,jj), 1 );
                blob_hues(2,blob_count+i) = ref_colors( LabelMatrix(ii,jj), 2 );
                blob_hues(3,blob_count+i) = ref_colors( LabelMatrix(ii,jj), 3 );

                blob_area(blob_count+i) = TArea(i);
                blob_bbox(blob_count+i) = TBBox(i);
                blob_major_axis(blob_count+i) = TMajorAxis(i);
                blob_minor_axis(blob_count+i) = TMinorAxis(i);
                blob_eccentricity(blob_count+i) = TEccent(i);
                blob_extent(blob_count+i) = TExtent(i);
                blob_orientation(blob_count+i) = TOrientation(i);
                
                blob_color(blob_count+i) = current_color;

            end
        end

        blob_count = blob_count + double(TNumBlobs);

    end
    
end


return

== matlab function Blob_Analysis/Blob_Analysis/IterativeSegmentation/Low Pass Filter/Low Pass Filter ==
  data: I input double; Iout output double
function Iout = GaussianBlurr(I)
% This function calculates the gaussian blur of an intensity image

sigma = sqrt(2);

Grows = 3;    % Gaussian matrix rows
Gcols = 3;    % Gaussian matrix columns

[Irows Icols] = size(I);

Iout = double(zeros(Irows,Icols));

Trows = Irows - Grows + 1;
Tcols = Icols - Gcols + 1;
Itemp = double(zeros(Trows,Tcols));

G = zeros(Grows,Gcols);

FirstRow = ceil(-Grows/2);
LastRow = floor(Grows/2);
FirstCol = ceil(-Gcols/2);
LastCol = floor(Gcols/2);
Gsum = 0;
for i=FirstRow:LastRow
    for j = FirstCol:LastCol
        G(i-FirstRow+1,j-FirstCol+1) = exp(-(j*j+i*i)/(2*sigma*sigma));
        Gsum = Gsum + G(i-FirstRow+1,j-FirstCol+1);
    end
end

G = G./Gsum;

Itemp = conv2(double(I),double(G),'valid');

% reflect boundaries to keep image the same size
% top
Iout((1:LastRow),(LastCol+1:Icols-LastCol)) = Itemp((1:LastRow),(1:Tcols));
% bottom
Iout((Irows-LastRow+1:Irows),(LastCol+1:Icols-LastCol)) = Itemp((Trows-LastRow+1:Trows),(1:Tcols));
% left
Iout((1+LastRow:Irows-LastRow),(1:LastCol)) = Itemp((1:Trows),(1:LastCol));
% right
Iout((1+LastRow:Irows-LastRow),(Icols-LastCol+1:Icols)) = Itemp((1:Trows),(Tcols-LastCol+1:Tcols));
% center
Iout((1+LastRow:Irows-LastRow),(1+LastCol:Icols-LastCol)) = Itemp;
% top left corner
Iout(1:LastRow,1:LastCol) = Itemp(1:LastRow,1:LastCol);
% top right corner
Iout(1:LastRow,Icols-LastCol:Icols) = Itemp(1:LastRow,Tcols-LastCol:Tcols);
% bottom left corner
Iout(Irows-LastRow:Irows,1:LastCol) = Itemp(Trows-LastRow:Trows,1:LastCol);
% bottom right corner
Iout(Irows-LastRow:Irows,Icols-LastCol:Icols) = Itemp(Trows-LastRow:Trows,Tcols-LastCol:Tcols);

return

== matlab function Blob_Analysis/Blob_Analysis/IterativeSegmentation/Low Pass Filter/Low Pass Filter1 ==
  data: I input double; Iout output double
function Iout = GaussianBlurr(I)
% This function calculates the gaussian blur of an intensity image

sigma = sqrt(2);

Grows = 3;    % Gaussian matrix rows
Gcols = 3;    % Gaussian matrix columns

[Irows Icols] = size(I);

Iout = double(zeros(Irows,Icols));

Trows = Irows - Grows + 1;
Tcols = Icols - Gcols + 1;
Itemp = double(zeros(Trows,Tcols));

G = zeros(Grows,Gcols);

FirstRow = ceil(-Grows/2);
LastRow = floor(Grows/2);
FirstCol = ceil(-Gcols/2);
LastCol = floor(Gcols/2);
Gsum = 0;
for i=FirstRow:LastRow
    for j = FirstCol:LastCol
        G(i-FirstRow+1,j-FirstCol+1) = exp(-(j*j+i*i)/(2*sigma*sigma));
        Gsum = Gsum + G(i-FirstRow+1,j-FirstCol+1);
    end
end

G = G./Gsum;

Itemp = conv2(double(I),double(G),'valid');

% reflect boundaries to keep image the same size
% top
Iout((1:LastRow),(LastCol+1:Icols-LastCol)) = Itemp((1:LastRow),(1:Tcols));
% bottom
Iout((Irows-LastRow+1:Irows),(LastCol+1:Icols-LastCol)) = Itemp((Trows-LastRow+1:Trows),(1:Tcols));
% left
Iout((1+LastRow:Irows-LastRow),(1:LastCol)) = Itemp((1:Trows),(1:LastCol));
% right
Iout((1+LastRow:Irows-LastRow),(Icols-LastCol+1:Icols)) = Itemp((1:Trows),(Tcols-LastCol+1:Tcols));
% center
Iout((1+LastRow:Irows-LastRow),(1+LastCol:Icols-LastCol)) = Itemp;
% top left corner
Iout(1:LastRow,1:LastCol) = Itemp(1:LastRow,1:LastCol);
% top right corner
Iout(1:LastRow,Icols-LastCol:Icols) = Itemp(1:LastRow,Tcols-LastCol:Tcols);
% bottom left corner
Iout(Irows-LastRow:Irows,1:LastCol) = Itemp(Trows-LastRow:Trows,1:LastCol);
% bottom right corner
Iout(Irows-LastRow:Irows,Icols-LastCol:Icols) = Itemp(Trows-LastRow:Trows,Tcols-LastCol:Tcols);

return

== matlab function Blob_Analysis/Blob_Analysis/IterativeSegmentation/Low Pass Filter/Low Pass Filter2 ==
  data: I input double; Iout output double
function Iout = GaussianBlurr(I)
% This function calculates the gaussian blur of an intensity image

sigma = sqrt(2);

Grows = 3;    % Gaussian matrix rows
Gcols = 3;    % Gaussian matrix columns

[Irows Icols] = size(I);

Iout = double(zeros(Irows,Icols));

Trows = Irows - Grows + 1;
Tcols = Icols - Gcols + 1;
Itemp = double(zeros(Trows,Tcols));

G = zeros(Grows,Gcols);

FirstRow = ceil(-Grows/2);
LastRow = floor(Grows/2);
FirstCol = ceil(-Gcols/2);
LastCol = floor(Gcols/2);
Gsum = 0;
for i=FirstRow:LastRow
    for j = FirstCol:LastCol
        G(i-FirstRow+1,j-FirstCol+1) = exp(-(j*j+i*i)/(2*sigma*sigma));
        Gsum = Gsum + G(i-FirstRow+1,j-FirstCol+1);
    end
end

G = G./Gsum;

Itemp = conv2(double(I),double(G),'valid');

% reflect boundaries to keep image the same size
% top
Iout((1:LastRow),(LastCol+1:Icols-LastCol)) = Itemp((1:LastRow),(1:Tcols));
% bottom
Iout((Irows-LastRow+1:Irows),(LastCol+1:Icols-LastCol)) = Itemp((Trows-LastRow+1:Trows),(1:Tcols));
% left
Iout((1+LastRow:Irows-LastRow),(1:LastCol)) = Itemp((1:Trows),(1:LastCol));
% right
Iout((1+LastRow:Irows-LastRow),(Icols-LastCol+1:Icols)) = Itemp((1:Trows),(Tcols-LastCol+1:Tcols));
% center
Iout((1+LastRow:Irows-LastRow),(1+LastCol:Icols-LastCol)) = Itemp;
% top left corner
Iout(1:LastRow,1:LastCol) = Itemp(1:LastRow,1:LastCol);
% top right corner
Iout(1:LastRow,Icols-LastCol:Icols) = Itemp(1:LastRow,Tcols-LastCol:Tcols);
% bottom left corner
Iout(Irows-LastRow:Irows,1:LastCol) = Itemp(Trows-LastRow:Trows,1:LastCol);
% bottom right corner
Iout(Irows-LastRow:Irows,Icols-LastCol:Icols) = Itemp(Trows-LastRow:Trows,Tcols-LastCol:Tcols);

return

== matlab function Blob_Analysis/Blob_Analysis/IterativeSegmentation/Segmentation/LabSegmentation ==
  data: L input double; LabelMatrix output double; a input double; b input double; ref_colors input double; num_colors input double
function LabelMatrix  = LabSegmentation(L,a,b,ref_colors,num_colors)
% This function generates the label matrix

[rows cols] = size(L);
LabelMatrix = zeros(rows,cols);

for i = 1:rows
    for j = 1:cols
        min_dist = 1000;
        index = 1;
        for k = 1:num_colors
            dist = sqrt((ref_colors(k,1) - L(i,j))^2 + (ref_colors(k,2) - a(i,j))^2 + (ref_colors(k,3) - b(i,j))^2);
            if(dist < min_dist)
                min_dist = double(dist);
                index = k;
            end
        end
        LabelMatrix(i,j) = index;
    end
end


return

== matlab function Blob_Analysis/Blob_Analysis/IterativeSegmentation/Segmentation/Reference Color Selection ==
  data: L input double; ref_colors output double; a input double; b input double; num_colors output double; Dist_Thresh input double
function [ref_colors, num_colors] = Segmentation(L,a,b,Dist_Thresh)
% This function tries segmentation by adding new reference colors everytime
% a pixel is found with a distance greater than a certain amount from
% every other reference color

[rows cols] = size(L);

Dist_Threshold = Dist_Thresh;% L = 0 to 100, a = -100 to 100, b = -100 to 100
                    % max dist = 300 -> 60/300 is 20%
x = 1;  % coefficients determining distance calculation
y = 1.5;
z = 1.5;

max_num_colors = 50;
ref_colors = zeros(max_num_colors,3);   % At most 50 different reference colors
LabelMatrix = zeros(rows,cols);
num_colors = 1;

center_row = floor(rows/2);
center_col = floor(cols/2);

% Define first reference color to be colr
ref_colors(1,:) = [L(center_row,center_col) a(center_row,center_col) b(center_row,center_col)];

flag = 0;
i = 1;
j = 1;
while(i <= rows)        % perform initial segmentation
    while(i <= rows && flag == 0)
        while(j <= cols && flag == 0)
            k = 1;
            min_dist = 1000;
            index = 1;
            while(k <= num_colors)
                dist = sqrt(x*(ref_colors(k,1) - L(i,j))^2 + y*(ref_colors(k,2) - a(i,j))^2 + z*(ref_colors(k,3) - b(i,j))^2);
                if(min_dist > dist)
                    min_dist = double(dist);
                    index = k;
                end
                k = k + 1;
            end
            if(j == 117)
                cow = 1;
            end
            if(min_dist > Dist_Threshold && num_colors < max_num_colors)
                ref_colors(num_colors+1,:) = [L(i,j) a(i,j) b(i,j)];
                num_colors = num_colors + 1;
                flag = 1;
                i = 0;
                j = 0;
            else
                LabelMatrix(i,j) = index;
            end
            j = j + 1;
        end
        j = 1;
        i = i + 1;
    end
    flag = 0;
end

% Go through image once more to get more accurate values for the different regions
ref_color_L_avg = zeros(50,1);
ref_color_a_avg = zeros(50,1);
ref_color_b_avg = zeros(50,1);
color_count = zeros(50,1);
for i = 1:rows
    for j = 1:cols
        index = LabelMatrix(i,j);
        ref_color_L_avg(index) = ref_color_L_avg(index) + L(i,j);
        ref_color_a_avg(index) = ref_color_a_avg(index) + a(i,j);
        ref_color_b_avg(index) = ref_color_b_avg(index) + b(i,j);
        color_count(index) = color_count(index) + 1;
    end
end
ref_color_L_avg = ref_color_L_avg ./ color_count;
ref_color_a_avg = ref_color_a_avg ./ color_count;
ref_color_b_avg = ref_color_b_avg ./ color_count;

for i = 1:num_colors
    ref_colors(i,1) = ref_color_L_avg(i);
    ref_colors(i,2) = ref_color_a_avg(i);
    ref_colors(i,3) = ref_color_b_avg(i);
end

return

== matlab function Blob_Analysis/Blob_Analysis/Segmented Image/Display Image ==
  data: LabelMatrix input double; ref_colors input double; L output double; a output double; b output double
function [L, a, b] = Display_Image(LabelMatrix, ref_colors)


% Initialize
[rows,cols] = size(LabelMatrix);
L = zeros(rows,cols);
a = zeros(rows,cols);
b = zeros(rows,cols);


% Allow only colors in specified range
for r = 1:rows
    for c = 1:cols
        
        L(r,c) = ref_colors(LabelMatrix(r,c), 1);
        a(r,c) = ref_colors(LabelMatrix(r,c), 2);
        b(r,c) = ref_colors(LabelMatrix(r,c), 3);
        
    end
end


return
